simulink model "Timon"  (R2020a)
settings: Solver=VariableStepAuto  StartTime=0.0  StopTime=10.0  RelTol=1e-3
libraries: simulink x1
settings Model: Creator=micro microndas  LastModifiedBy=micro microndas

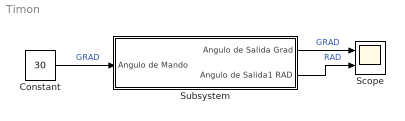
== system Timon ==
  Constant : Constant  Value=30
  Scope : Scope  NumInputPorts=2
  Subsystem : Subsystem
  wires:
  Constant/1 -> Subsystem/1(Angulo de Mando)  "GRAD"
  Subsystem/1(Angulo de Salida Grad) -> Scope/1  "GRAD"
  Subsystem/2(Angulo de Salida1 RAD) -> Scope/2  "RAD"

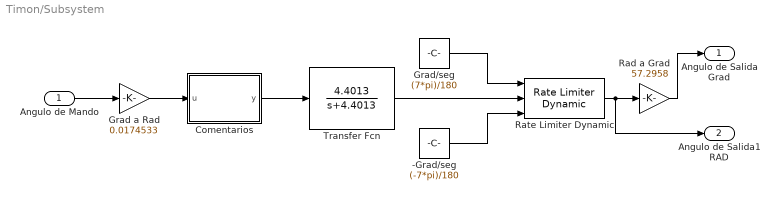
== system Timon/Subsystem ==
  Angulo de Mando : Inport
  -Grad/seg : Constant  Value=(-7*pi)/180
  Comentarios : MATLAB Function  TreatAsAtomicUnit=on
  Grad a Rad : Gain  Gain=0.0174533
  Grad/seg : Constant  Value=(7*pi)/180
  Rad a Grad : Gain  Gain=57.2958
  Rate Limiter Dynamic : simulink/Discontinuities/Rate Limiter Dynamic
  Transfer Fcn : TransferFcn  Numerator=[4.4013]  Denominator=[1 4.4013]
  Angulo de Salida Grad : Outport
  Angulo de Salida1 RAD : Outport  Port=2
  wires:
  Transfer Fcn/1 -> Rate Limiter Dynamic/2
  Grad/seg/1 -> Rate Limiter Dynamic/1
  -Grad/seg/1 -> Rate Limiter Dynamic/3
  Angulo de Mando/1 -> Grad a Rad/1
  Rate Limiter Dynamic/1 -> Angulo de Salida1 RAD/1, Rad a Grad/1
  Rad a Grad/1 -> Angulo de Salida Grad/1
  Grad a Rad/1 -> Comentarios/1(u)
  Comentarios/1(y) -> Transfer Fcn/1

== matlab function Timon/Subsystem/Comentarios ==
  data: u input; y output
function y = fcn(u)

%Kg' = Kg*L / U
    %Kg = Maximo giro del timon / error maximo
        %error maximo
        %Maximo giro del timon
    %L = Eslora / Longitud del buque
        %390.00 𝑓𝑡 
        %118.872 mts
    %U = Velocidad del buque
        %15 nudo nautico
        %7.7166 m/s

y = u;
